simulink model "TST_FlSys_FlCons"  (R2016b)
settings: Solver=FixedStepDiscrete  StartTime=0.0  StopTime=1  FixedStep=sampleTime  RelTol=1e-3
values from neighbouring files (symbols this model uses):
  testCase = 1    [initTST_FlSys_FlCons_001.m]    (also in initTST_FlSys_FlCons_002.m = 2)
libraries: simulink x9, UnitTest_Lib x6
settings Model: Creator=zhengjinyan  LastModifiedBy=zhengjinyan
settings DebuggingCC: SignalRangeChecking=error

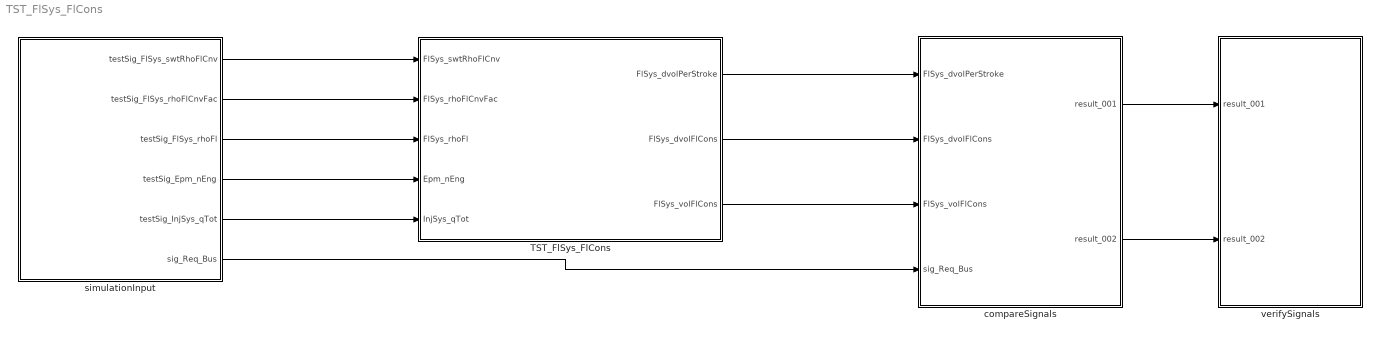
== system TST_FlSys_FlCons ==
  TST_FlSys_FlCons : Subsystem
  compareSignals : Subsystem
  simulationInput : Subsystem
  verifySignals : Subsystem
  wires:
  simulationInput/1(testSig_FlSys_swtRhoFlCnv) -> TST_FlSys_FlCons/1(FlSys_swtRhoFlCnv)
  simulationInput/2(testSig_FlSys_rhoFlCnvFac) -> TST_FlSys_FlCons/2(FlSys_rhoFlCnvFac)
  simulationInput/3(testSig_FlSys_rhoFl) -> TST_FlSys_FlCons/3(FlSys_rhoFl)
  simulationInput/4(testSig_Epm_nEng) -> TST_FlSys_FlCons/4(Epm_nEng)
  simulationInput/5(testSig_InjSys_qTot) -> TST_FlSys_FlCons/5(InjSys_qTot)
  TST_FlSys_FlCons/1(FlSys_dvolPerStroke) -> compareSignals/1(FlSys_dvolPerStroke)
  TST_FlSys_FlCons/2(FlSys_dvolFlCons) -> compareSignals/2(FlSys_dvolFlCons)
  TST_FlSys_FlCons/3(FlSys_volFlCons) -> compareSignals/3(FlSys_volFlCons)
  simulationInput/6(sig_Req_Bus) -> compareSignals/4(sig_Req_Bus)
  compareSignals/1(result_001) -> verifySignals/1(result_001)
  compareSignals/2(result_002) -> verifySignals/2(result_002)

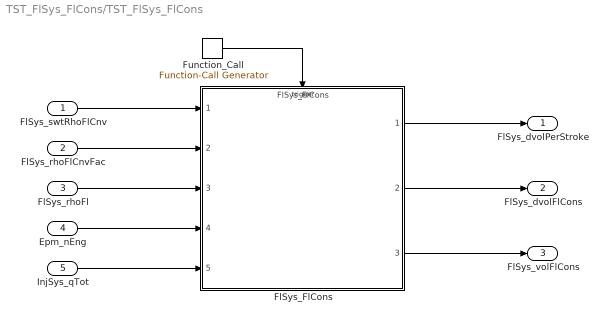
== system TST_FlSys_FlCons/TST_FlSys_FlCons ==
  FlSys_swtRhoFlCnv : Inport
  FlSys_rhoFlCnvFac : Inport  Port=2
  FlSys_rhoFl : Inport  Port=3
  Epm_nEng : Inport  Port=4
  InjSys_qTot : Inport  Port=5
  FlSys_FlCons : ModelReference  ModelNameDialog=FlSys_FlCons  SimulationMode=Normal  ModelReferenceVersion=1.6  TriggerPortName=function  TriggerPortTriggerType=function-call  TriggerPortStatesWhenEnabling=held
  Function_Call : simulink/Ports & Subsystems/Function-Call Generator  sample_time=sampleTime  numberOfIterations=1
  FlSys_dvolPerStroke : Outport
  FlSys_dvolFlCons : Outport  Port=2
  FlSys_volFlCons : Outport  Port=3
  wires:
  Function_Call/1 -> FlSys_FlCons/Trigger
  FlSys_swtRhoFlCnv/1 -> FlSys_FlCons/1
  FlSys_rhoFlCnvFac/1 -> FlSys_FlCons/2
  FlSys_rhoFl/1 -> FlSys_FlCons/3
  Epm_nEng/1 -> FlSys_FlCons/4
  InjSys_qTot/1 -> FlSys_FlCons/5
  FlSys_FlCons/1 -> FlSys_dvolPerStroke/1
  FlSys_FlCons/2 -> FlSys_dvolFlCons/1
  FlSys_FlCons/3 -> FlSys_volFlCons/1

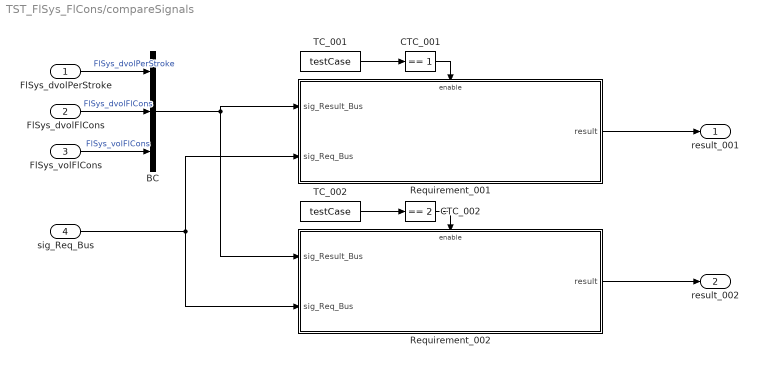
== system TST_FlSys_FlCons/compareSignals ==
  FlSys_dvolPerStroke : Inport
  FlSys_dvolFlCons : Inport  Port=2
  FlSys_volFlCons : Inport  Port=3
  sig_Req_Bus : Inport  Port=4
  BC : BusCreator  Inputs=3
  CTC_001 : simulink/Logic and Bit Operations/Compare To Constant  relop===  const=1  OutDataTypeStr=boolean
  CTC_002 : simulink/Logic and Bit Operations/Compare To Constant  relop===  const=2  OutDataTypeStr=boolean
  Requirement_001 : Subsystem
  Requirement_002 : Subsystem
  TC_001 : Constant  Value=testCase
  TC_002 : Constant  Value=testCase
  result_001 : Outport
  result_002 : Outport  Port=2
  wires:
  FlSys_dvolPerStroke/1 -> BC/1  "FlSys_dvolPerStroke"
  FlSys_dvolFlCons/1 -> BC/2  "FlSys_dvolFlCons"
  FlSys_volFlCons/1 -> BC/3  "FlSys_volFlCons"
  TC_001/1 -> CTC_001/1
  CTC_001/1 -> Requirement_001/Enable
  sig_Req_Bus/1 -> Requirement_001/2(sig_Req_Bus), Requirement_002/2(sig_Req_Bus)
  BC/1 -> Requirement_001/1(sig_Result_Bus), Requirement_002/1(sig_Result_Bus)
  Requirement_001/1(result) -> result_001/1
  TC_002/1 -> CTC_002/1
  CTC_002/1 -> Requirement_002/Enable
  Requirement_002/1(result) -> result_002/1

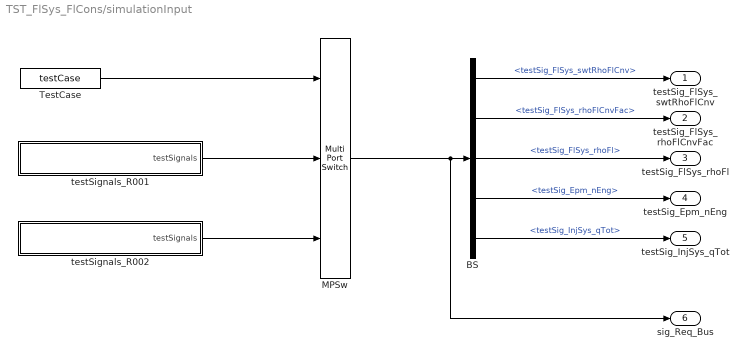
== system TST_FlSys_FlCons/simulationInput ==
  BS : BusSelector  OutputSignals=testSig_FlSys_swtRhoFlCnv,testSig_FlSys_rhoFlCnvFac,testSig_FlSys_rhoFl,testSig_Epm_nEng,testSig_InjSys_qTot
  MPSw : MultiPortSwitch  Inputs=2  SaturateOnIntegerOverflow=on  InputSameDT=on
  TestCase : Constant  Value=testCase
  testSignals_R001 : Subsystem
  testSignals_R002 : Subsystem
  testSig_FlSys_swtRhoFlCnv : Outport
  testSig_FlSys_rhoFlCnvFac : Outport  Port=2
  testSig_FlSys_rhoFl : Outport  Port=3
  testSig_Epm_nEng : Outport  Port=4
  testSig_InjSys_qTot : Outport  Port=5
  sig_Req_Bus : Outport  Port=6
  wires:
  BS/1 -> testSig_FlSys_swtRhoFlCnv/1  "<testSig_FlSys_swtRhoFlCnv>"
  BS/2 -> testSig_FlSys_rhoFlCnvFac/1  "<testSig_FlSys_rhoFlCnvFac>"
  BS/3 -> testSig_FlSys_rhoFl/1  "<testSig_FlSys_rhoFl>"
  BS/4 -> testSig_Epm_nEng/1  "<testSig_Epm_nEng>"
  BS/5 -> testSig_InjSys_qTot/1  "<testSig_InjSys_qTot>"
  MPSw/1 -> BS/1, sig_Req_Bus/1
  TestCase/1 -> MPSw/1
  testSignals_R001/1(testSignals) -> MPSw/2
  testSignals_R002/1(testSignals) -> MPSw/3

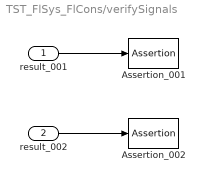
== system TST_FlSys_FlCons/verifySignals ==
  result_001 : Inport
  result_002 : Inport  Port=2
  Assertion_001 : Assertion  Enabled=off
  Assertion_002 : Assertion  Enabled=off
  wires:
  result_001/1 -> Assertion_001/1
  result_002/1 -> Assertion_002/1

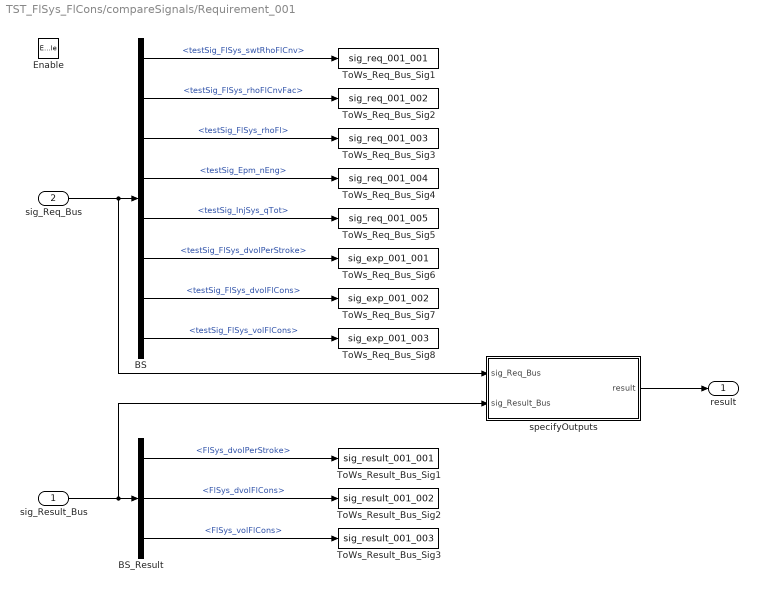
== system TST_FlSys_FlCons/compareSignals/Requirement_001 ==
  sig_Result_Bus : Inport
  sig_Req_Bus : Inport  Port=2
  Enable : EnablePort
  BS : BusSelector  OutputSignals=testSig_FlSys_swtRhoFlCnv,testSig_FlSys_rhoFlCnvFac,testSig_FlSys_rhoFl,testSig_Epm_nEng,testSig_InjSys_qTot,testSig_FlSys_dvolPerStroke,testSig_FlSys_dvolFlCons,testSig_FlSys_volFlCons
  BS_Result : BusSelector  OutputSignals=FlSys_dvolPerStroke,FlSys_dvolFlCons,FlSys_volFlCons
  ToWs_Req_Bus_Sig1 : ToWorkspace  VariableName=sig_req_001_001  SaveFormat=Structure With Time
  ToWs_Req_Bus_Sig2 : ToWorkspace  VariableName=sig_req_001_002  SaveFormat=Structure With Time
  ToWs_Req_Bus_Sig3 : ToWorkspace  VariableName=sig_req_001_003  SaveFormat=Structure With Time
  ToWs_Req_Bus_Sig4 : ToWorkspace  VariableName=sig_req_001_004  SaveFormat=Structure With Time
  ToWs_Req_Bus_Sig5 : ToWorkspace  VariableName=sig_req_001_005  SaveFormat=Structure With Time
  ToWs_Req_Bus_Sig6 : ToWorkspace  VariableName=sig_exp_001_001  SaveFormat=Structure With Time
  ToWs_Req_Bus_Sig7 : ToWorkspace  VariableName=sig_exp_001_002  SaveFormat=Structure With Time
  ToWs_Req_Bus_Sig8 : ToWorkspace  VariableName=sig_exp_001_003  SaveFormat=Structure With Time
  ToWs_Result_Bus_Sig1 : ToWorkspace  VariableName=sig_result_001_001  SaveFormat=Structure With Time
  ToWs_Result_Bus_Sig2 : ToWorkspace  VariableName=sig_result_001_002  SaveFormat=Structure With Time
  ToWs_Result_Bus_Sig3 : ToWorkspace  VariableName=sig_result_001_003  SaveFormat=Structure With Time
  specifyOutputs : Subsystem
  result : Outport
  wires:
  sig_Req_Bus/1 -> BS/1, specifyOutputs/1(sig_Req_Bus)
  BS/1 -> ToWs_Req_Bus_Sig1/1  "<testSig_FlSys_swtRhoFlCnv>"
  BS/2 -> ToWs_Req_Bus_Sig2/1  "<testSig_FlSys_rhoFlCnvFac>"
  BS/3 -> ToWs_Req_Bus_Sig3/1  "<testSig_FlSys_rhoFl>"
  BS/4 -> ToWs_Req_Bus_Sig4/1  "<testSig_Epm_nEng>"
  BS/5 -> ToWs_Req_Bus_Sig5/1  "<testSig_InjSys_qTot>"
  BS/6 -> ToWs_Req_Bus_Sig6/1  "<testSig_FlSys_dvolPerStroke>"
  BS/7 -> ToWs_Req_Bus_Sig7/1  "<testSig_FlSys_dvolFlCons>"
  BS/8 -> ToWs_Req_Bus_Sig8/1  "<testSig_FlSys_volFlCons>"
  sig_Result_Bus/1 -> BS_Result/1, specifyOutputs/2(sig_Result_Bus)
  BS_Result/1 -> ToWs_Result_Bus_Sig1/1  "<FlSys_dvolPerStroke>"
  BS_Result/2 -> ToWs_Result_Bus_Sig2/1  "<FlSys_dvolFlCons>"
  BS_Result/3 -> ToWs_Result_Bus_Sig3/1  "<FlSys_volFlCons>"
  specifyOutputs/1(result) -> result/1

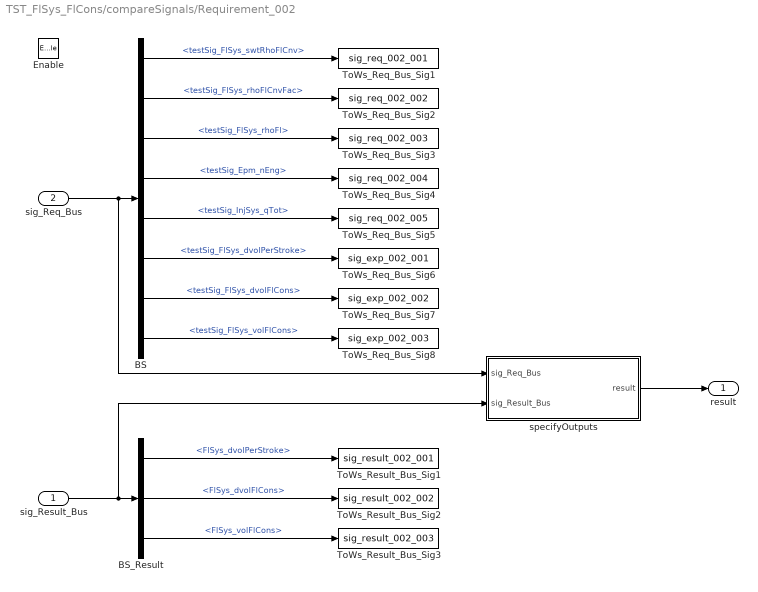
== system TST_FlSys_FlCons/compareSignals/Requirement_002 ==
  sig_Result_Bus : Inport
  sig_Req_Bus : Inport  Port=2
  Enable : EnablePort
  BS : BusSelector  OutputSignals=testSig_FlSys_swtRhoFlCnv,testSig_FlSys_rhoFlCnvFac,testSig_FlSys_rhoFl,testSig_Epm_nEng,testSig_InjSys_qTot,testSig_FlSys_dvolPerStroke,testSig_FlSys_dvolFlCons,testSig_FlSys_volFlCons
  BS_Result : BusSelector  OutputSignals=FlSys_dvolPerStroke,FlSys_dvolFlCons,FlSys_volFlCons
  ToWs_Req_Bus_Sig1 : ToWorkspace  VariableName=sig_req_002_001  SaveFormat=Structure With Time
  ToWs_Req_Bus_Sig2 : ToWorkspace  VariableName=sig_req_002_002  SaveFormat=Structure With Time
  ToWs_Req_Bus_Sig3 : ToWorkspace  VariableName=sig_req_002_003  SaveFormat=Structure With Time
  ToWs_Req_Bus_Sig4 : ToWorkspace  VariableName=sig_req_002_004  SaveFormat=Structure With Time
  ToWs_Req_Bus_Sig5 : ToWorkspace  VariableName=sig_req_002_005  SaveFormat=Structure With Time
  ToWs_Req_Bus_Sig6 : ToWorkspace  VariableName=sig_exp_002_001  SaveFormat=Structure With Time
  ToWs_Req_Bus_Sig7 : ToWorkspace  VariableName=sig_exp_002_002  SaveFormat=Structure With Time
  ToWs_Req_Bus_Sig8 : ToWorkspace  VariableName=sig_exp_002_003  SaveFormat=Structure With Time
  ToWs_Result_Bus_Sig1 : ToWorkspace  VariableName=sig_result_002_001  SaveFormat=Structure With Time
  ToWs_Result_Bus_Sig2 : ToWorkspace  VariableName=sig_result_002_002  SaveFormat=Structure With Time
  ToWs_Result_Bus_Sig3 : ToWorkspace  VariableName=sig_result_002_003  SaveFormat=Structure With Time
  specifyOutputs : Subsystem
  result : Outport
  wires:
  sig_Req_Bus/1 -> BS/1, specifyOutputs/1(sig_Req_Bus)
  BS/1 -> ToWs_Req_Bus_Sig1/1  "<testSig_FlSys_swtRhoFlCnv>"
  BS/2 -> ToWs_Req_Bus_Sig2/1  "<testSig_FlSys_rhoFlCnvFac>"
  BS/3 -> ToWs_Req_Bus_Sig3/1  "<testSig_FlSys_rhoFl>"
  BS/4 -> ToWs_Req_Bus_Sig4/1  "<testSig_Epm_nEng>"
  BS/5 -> ToWs_Req_Bus_Sig5/1  "<testSig_InjSys_qTot>"
  BS/6 -> ToWs_Req_Bus_Sig6/1  "<testSig_FlSys_dvolPerStroke>"
  BS/7 -> ToWs_Req_Bus_Sig7/1  "<testSig_FlSys_dvolFlCons>"
  BS/8 -> ToWs_Req_Bus_Sig8/1  "<testSig_FlSys_volFlCons>"
  sig_Result_Bus/1 -> BS_Result/1, specifyOutputs/2(sig_Result_Bus)
  BS_Result/1 -> ToWs_Result_Bus_Sig1/1  "<FlSys_dvolPerStroke>"
  BS_Result/2 -> ToWs_Result_Bus_Sig2/1  "<FlSys_dvolFlCons>"
  BS_Result/3 -> ToWs_Result_Bus_Sig3/1  "<FlSys_volFlCons>"
  specifyOutputs/1(result) -> result/1

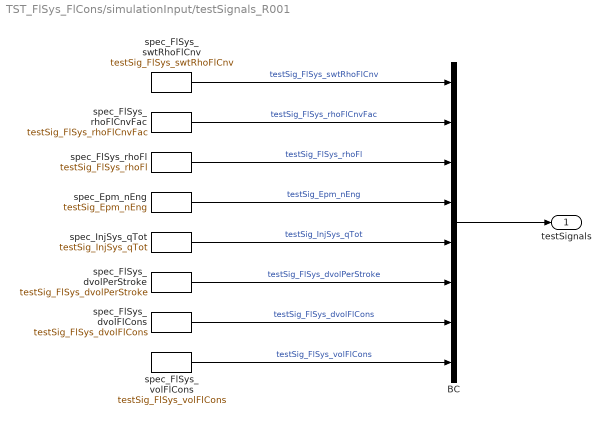
== system TST_FlSys_FlCons/simulationInput/testSignals_R001 ==
  BC : BusCreator  Inputs=8
  spec_Epm_nEng : FromWorkspace  VariableName=testSig_Epm_nEng  Interpolate=off  OutputAfterFinalValue=Holding final value
  spec_FlSys_dvolFlCons : FromWorkspace  VariableName=testSig_FlSys_dvolFlCons  Interpolate=off  OutputAfterFinalValue=Holding final value
  spec_FlSys_dvolPerStroke : FromWorkspace  VariableName=testSig_FlSys_dvolPerStroke  Interpolate=off  OutputAfterFinalValue=Holding final value
  spec_FlSys_rhoFl : FromWorkspace  VariableName=testSig_FlSys_rhoFl  Interpolate=off  OutputAfterFinalValue=Holding final value
  spec_FlSys_rhoFlCnvFac : FromWorkspace  VariableName=testSig_FlSys_rhoFlCnvFac  Interpolate=off  OutputAfterFinalValue=Holding final value
  spec_FlSys_swtRhoFlCnv : FromWorkspace  VariableName=testSig_FlSys_swtRhoFlCnv  Interpolate=off  OutputAfterFinalValue=Holding final value
  spec_FlSys_volFlCons : FromWorkspace  VariableName=testSig_FlSys_volFlCons  Interpolate=off  OutputAfterFinalValue=Holding final value
  spec_InjSys_qTot : FromWorkspace  VariableName=testSig_InjSys_qTot  Interpolate=off  OutputAfterFinalValue=Holding final value
  testSignals : Outport
  wires:
  BC/1 -> testSignals/1
  spec_FlSys_swtRhoFlCnv/1 -> BC/1  "testSig_FlSys_swtRhoFlCnv"
  spec_FlSys_rhoFlCnvFac/1 -> BC/2  "testSig_FlSys_rhoFlCnvFac"
  spec_FlSys_rhoFl/1 -> BC/3  "testSig_FlSys_rhoFl"
  spec_Epm_nEng/1 -> BC/4  "testSig_Epm_nEng"
  spec_InjSys_qTot/1 -> BC/5  "testSig_InjSys_qTot"
  spec_FlSys_dvolPerStroke/1 -> BC/6  "testSig_FlSys_dvolPerStroke"
  spec_FlSys_dvolFlCons/1 -> BC/7  "testSig_FlSys_dvolFlCons"
  spec_FlSys_volFlCons/1 -> BC/8  "testSig_FlSys_volFlCons"

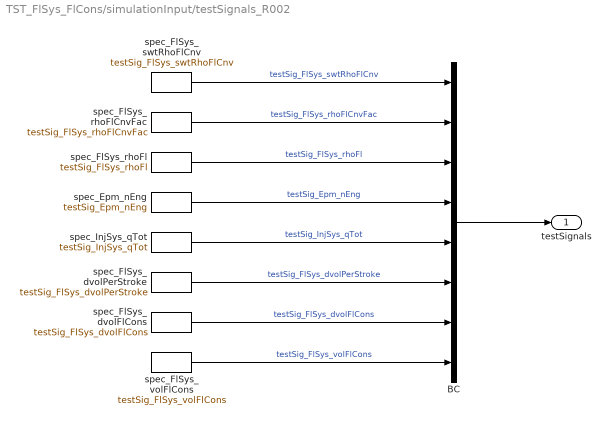
== system TST_FlSys_FlCons/simulationInput/testSignals_R002 ==
  BC : BusCreator  Inputs=8
  spec_Epm_nEng : FromWorkspace  VariableName=testSig_Epm_nEng  Interpolate=off  OutputAfterFinalValue=Holding final value
  spec_FlSys_dvolFlCons : FromWorkspace  VariableName=testSig_FlSys_dvolFlCons  Interpolate=off  OutputAfterFinalValue=Holding final value
  spec_FlSys_dvolPerStroke : FromWorkspace  VariableName=testSig_FlSys_dvolPerStroke  Interpolate=off  OutputAfterFinalValue=Holding final value
  spec_FlSys_rhoFl : FromWorkspace  VariableName=testSig_FlSys_rhoFl  Interpolate=off  OutputAfterFinalValue=Holding final value
  spec_FlSys_rhoFlCnvFac : FromWorkspace  VariableName=testSig_FlSys_rhoFlCnvFac  Interpolate=off  OutputAfterFinalValue=Holding final value
  spec_FlSys_swtRhoFlCnv : FromWorkspace  VariableName=testSig_FlSys_swtRhoFlCnv  Interpolate=off  OutputAfterFinalValue=Holding final value
  spec_FlSys_volFlCons : FromWorkspace  VariableName=testSig_FlSys_volFlCons  Interpolate=off  OutputAfterFinalValue=Holding final value
  spec_InjSys_qTot : FromWorkspace  VariableName=testSig_InjSys_qTot  Interpolate=off  OutputAfterFinalValue=Holding final value
  testSignals : Outport
  wires:
  BC/1 -> testSignals/1
  spec_FlSys_swtRhoFlCnv/1 -> BC/1  "testSig_FlSys_swtRhoFlCnv"
  spec_FlSys_rhoFlCnvFac/1 -> BC/2  "testSig_FlSys_rhoFlCnvFac"
  spec_FlSys_rhoFl/1 -> BC/3  "testSig_FlSys_rhoFl"
  spec_Epm_nEng/1 -> BC/4  "testSig_Epm_nEng"
  spec_InjSys_qTot/1 -> BC/5  "testSig_InjSys_qTot"
  spec_FlSys_dvolPerStroke/1 -> BC/6  "testSig_FlSys_dvolPerStroke"
  spec_FlSys_dvolFlCons/1 -> BC/7  "testSig_FlSys_dvolFlCons"
  spec_FlSys_volFlCons/1 -> BC/8  "testSig_FlSys_volFlCons"

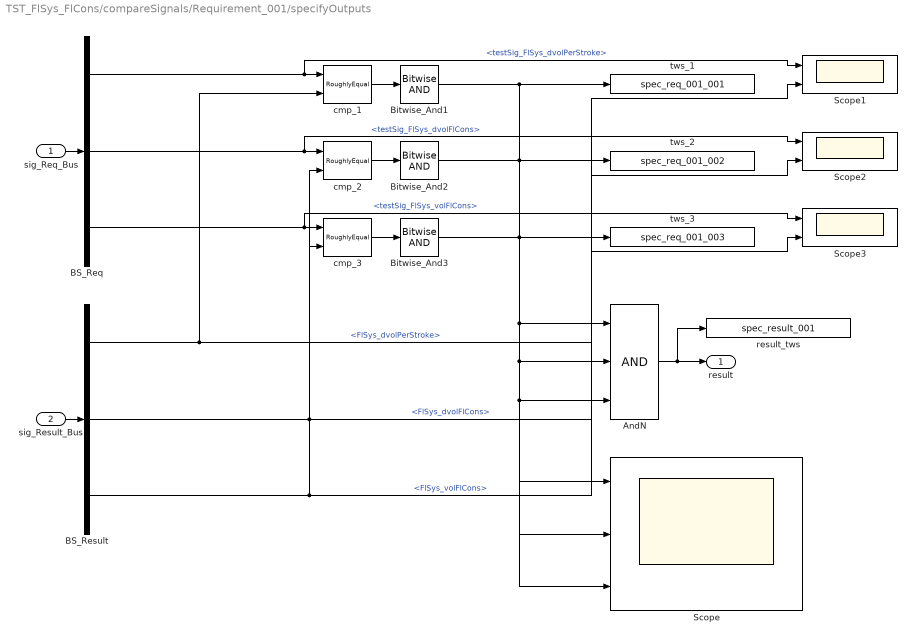
== system TST_FlSys_FlCons/compareSignals/Requirement_001/specifyOutputs ==
  sig_Req_Bus : Inport
  sig_Result_Bus : Inport  Port=2
  AndN : Logic  Inputs=3
  BS_Req : BusSelector  OutputSignals=testSig_FlSys_dvolPerStroke,testSig_FlSys_dvolFlCons,testSig_FlSys_volFlCons
  BS_Result : BusSelector  OutputSignals=FlSys_dvolPerStroke,FlSys_dvolFlCons,FlSys_volFlCons
  Bitwise_And1 : simulink/Logic and Bit Operations/Bitwise Operator  logicop=AND  UseBitMask=off  BitMask=bin2dec('11011001')  BitMaskRealWorld=Stored Integer
  Bitwise_And2 : simulink/Logic and Bit Operations/Bitwise Operator  logicop=AND  UseBitMask=off  BitMask=bin2dec('11011001')  BitMaskRealWorld=Stored Integer
  Bitwise_And3 : simulink/Logic and Bit Operations/Bitwise Operator  logicop=AND  UseBitMask=off  BitMask=bin2dec('11011001')  BitMaskRealWorld=Stored Integer
  Scope : Scope  NumInputPorts=3
  Scope1 : Scope  NumInputPorts=2
  Scope2 : Scope  NumInputPorts=2
  Scope3 : Scope  NumInputPorts=2
  cmp_1 : UnitTest_Lib/RoughlyEqual  slope=10
  cmp_2 : UnitTest_Lib/RoughlyEqual  slope=10
  cmp_3 : UnitTest_Lib/RoughlyEqual  slope=10
  result_tws : ToWorkspace  VariableName=spec_result_001
  tws_1 : ToWorkspace  VariableName=spec_req_001_001
  tws_2 : ToWorkspace  VariableName=spec_req_001_002
  tws_3 : ToWorkspace  VariableName=spec_req_001_003
  result : Outport
  wires:
  sig_Req_Bus/1 -> BS_Req/1
  sig_Result_Bus/1 -> BS_Result/1
  AndN/1 -> result/1, result_tws/1
  BS_Req/1 -> cmp_1/1, Scope1/1  "<testSig_FlSys_dvolPerStroke>"
  BS_Result/1 -> cmp_1/2, Scope1/2  "<FlSys_dvolPerStroke>"
  cmp_1/1 -> Bitwise_And1/1
  Bitwise_And1/1 -> AndN/1, Scope/1, tws_1/1
  BS_Req/2 -> cmp_2/1, Scope2/1  "<testSig_FlSys_dvolFlCons>"
  BS_Result/2 -> cmp_2/2, Scope2/2  "<FlSys_dvolFlCons>"
  cmp_2/1 -> Bitwise_And2/1
  Bitwise_And2/1 -> AndN/2, Scope/2, tws_2/1
  BS_Req/3 -> cmp_3/1, Scope3/1  "<testSig_FlSys_volFlCons>"
  BS_Result/3 -> cmp_3/2, Scope3/2  "<FlSys_volFlCons>"
  cmp_3/1 -> Bitwise_And3/1
  Bitwise_And3/1 -> AndN/3, Scope/3, tws_3/1

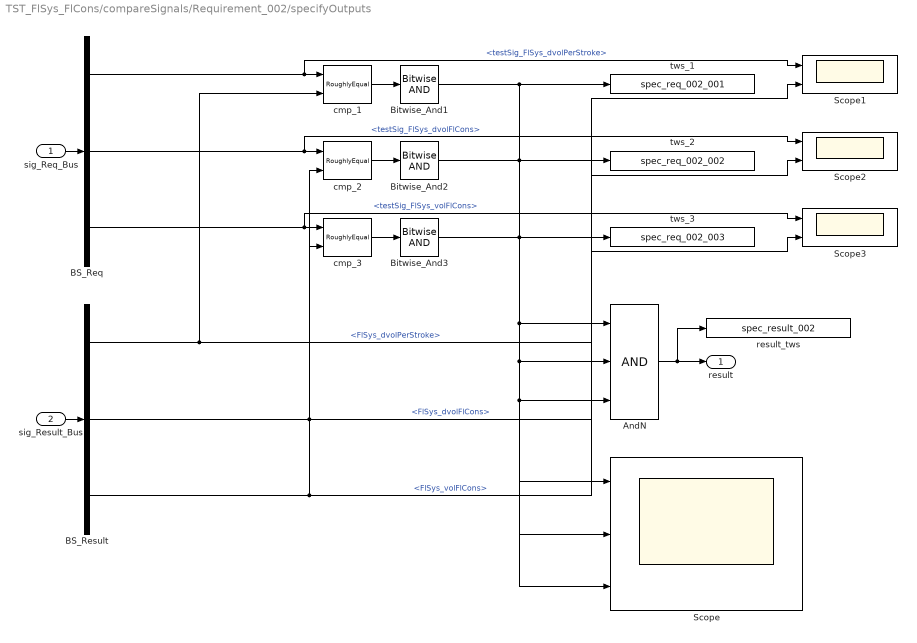
== system TST_FlSys_FlCons/compareSignals/Requirement_002/specifyOutputs ==
  sig_Req_Bus : Inport
  sig_Result_Bus : Inport  Port=2
  AndN : Logic  Inputs=3
  BS_Req : BusSelector  OutputSignals=testSig_FlSys_dvolPerStroke,testSig_FlSys_dvolFlCons,testSig_FlSys_volFlCons
  BS_Result : BusSelector  OutputSignals=FlSys_dvolPerStroke,FlSys_dvolFlCons,FlSys_volFlCons
  Bitwise_And1 : simulink/Logic and Bit Operations/Bitwise Operator  logicop=AND  UseBitMask=off  BitMask=bin2dec('11011001')  BitMaskRealWorld=Stored Integer
  Bitwise_And2 : simulink/Logic and Bit Operations/Bitwise Operator  logicop=AND  UseBitMask=off  BitMask=bin2dec('11011001')  BitMaskRealWorld=Stored Integer
  Bitwise_And3 : simulink/Logic and Bit Operations/Bitwise Operator  logicop=AND  UseBitMask=off  BitMask=bin2dec('11011001')  BitMaskRealWorld=Stored Integer
  Scope : Scope  NumInputPorts=3
  Scope1 : Scope  NumInputPorts=2
  Scope2 : Scope  NumInputPorts=2
  Scope3 : Scope  NumInputPorts=2
  cmp_1 : UnitTest_Lib/RoughlyEqual  slope=10
  cmp_2 : UnitTest_Lib/RoughlyEqual  slope=10
  cmp_3 : UnitTest_Lib/RoughlyEqual  slope=10
  result_tws : ToWorkspace  VariableName=spec_result_002
  tws_1 : ToWorkspace  VariableName=spec_req_002_001
  tws_2 : ToWorkspace  VariableName=spec_req_002_002
  tws_3 : ToWorkspace  VariableName=spec_req_002_003
  result : Outport
  wires:
  sig_Req_Bus/1 -> BS_Req/1
  sig_Result_Bus/1 -> BS_Result/1
  AndN/1 -> result/1, result_tws/1
  BS_Req/1 -> cmp_1/1, Scope1/1  "<testSig_FlSys_dvolPerStroke>"
  BS_Result/1 -> cmp_1/2, Scope1/2  "<FlSys_dvolPerStroke>"
  cmp_1/1 -> Bitwise_And1/1
  Bitwise_And1/1 -> AndN/1, Scope/1, tws_1/1
  BS_Req/2 -> cmp_2/1, Scope2/1  "<testSig_FlSys_dvolFlCons>"
  BS_Result/2 -> cmp_2/2, Scope2/2  "<FlSys_dvolFlCons>"
  cmp_2/1 -> Bitwise_And2/1
  Bitwise_And2/1 -> AndN/2, Scope/2, tws_2/1
  BS_Req/3 -> cmp_3/1, Scope3/1  "<testSig_FlSys_volFlCons>"
  BS_Result/3 -> cmp_3/2, Scope3/2  "<FlSys_volFlCons>"
  cmp_3/1 -> Bitwise_And3/1
  Bitwise_And3/1 -> AndN/3, Scope/3, tws_3/1
